simulink model "ex5"  (R2020a)
settings: Solver=VariableStepAuto  StartTime=0.0  StopTime=10.0  RelTol=1e-3
settings Model: Creator=Kundan Patil  LastModifiedBy=Kundan Patil

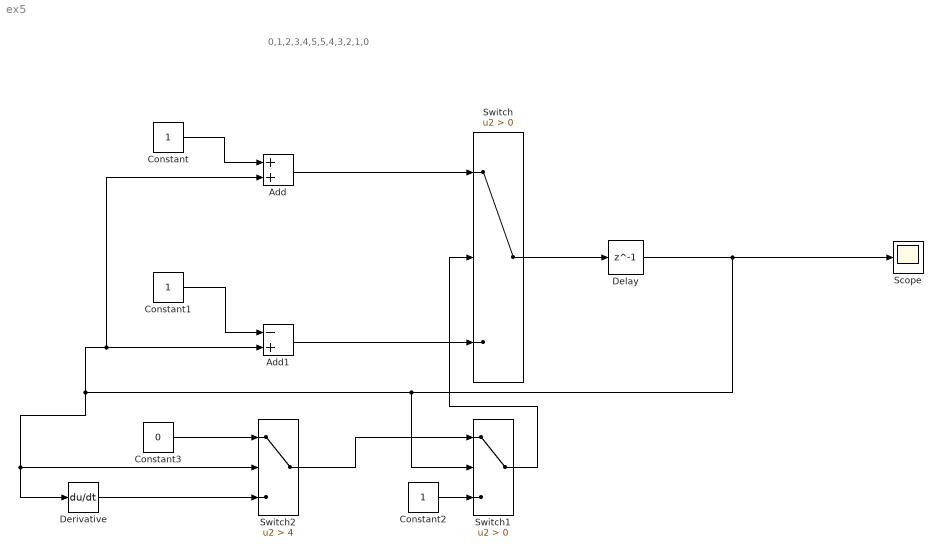
== system ex5 ==
  note: 0,1,2,3,4,5,5,4,3,2,1,0
  Add : Sum
  Add1 : Sum  Inputs=-+
  Constant : Constant
  Constant1 : Constant
  Constant2 : Constant
  Constant3 : Constant  Value=0
  Delay : Delay  DelayLength=1
  Derivative : Derivative
  Scope : Scope
  Switch : Switch  Criteria=u2 > Threshold
  Switch1 : Switch  Criteria=u2 > Threshold
  Switch2 : Switch  Criteria=u2 > Threshold  Threshold=4
  wires:
  Constant/1 -> Add/1
  Add/1 -> Switch/1
  Constant1/1 -> Add1/1
  Add1/1 -> Switch/3
  Delay/1 -> Derivative/1, Switch2/2, Add1/2, Add/2, Switch1/2, Scope/1
  Switch/1 -> Delay/1
  Constant2/1 -> Switch1/3
  Switch1/1 -> Switch/2
  Constant3/1 -> Switch2/1
  Derivative/1 -> Switch2/3
  Switch2/1 -> Switch1/1
